simulink model "sistema_temas_3y4"  (Simulink 8.6)
settings: Solver=FixedStepDiscrete  StartTime=0.0  StopTime=1000  RelTol=1e-3
libraries: libreria_temas_3y4 x2
settings Model: Creator=AJA  LastModifiedBy=Shagai
settings OptimizationCC: InitFltsAndDblsToZero=on
settings DebuggingCC: FcnCallInpInsideContextMsg=UseLocalSettings
settings HardwareCC: TargetHWDeviceType=32-bit Generic
settings GRTTargetCC: TargetFcnLib=ansi_tfl_tmw.mat

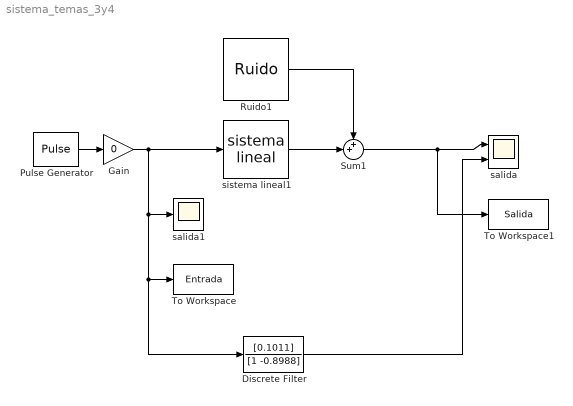
== system sistema_temas_3y4 ==
  Discrete Filter : DiscreteFilter  Numerator=[0.1011]  Denominator=[1 -0.8988]
  Gain : Gain  Gain=0
  Pulse Generator : DiscretePulseGenerator  Amplitude=80  Period=200  PulseWidth=100  SampleTime=0.1
  Ruido1 : libreria_temas_3y4/Ruido
  Sum1 : Sum  Inputs=++|
  To Workspace : ToWorkspace  VariableName=Entrada  SaveFormat=Timeseries  SampleTime=-1
  To Workspace1 : ToWorkspace  VariableName=Salida  SaveFormat=Timeseries  SampleTime=-1
  salida : Scope  NumInputPorts=2
  salida1 : Scope
  sistema lineal1 : libreria_temas_3y4/sistema lineal
  wires:
  Sum1/1 -> To Workspace1/1, salida/1
  Pulse Generator/1 -> Gain/1
  sistema lineal1/1 -> Sum1/2
  Gain/1 -> Discrete Filter/1, To Workspace/1, salida1/1, sistema lineal1/1
  Discrete Filter/1 -> salida/2
  Ruido1/1 -> Sum1/1
